simulink model "PID_CorSys_Ctrl"  (R2018b)
settings: Solver=ode1  StartTime=0.0  StopTime=inf  FixedStep=0.01  RelTol=1e-3  EnableMultiTasking=on
libraries: gtbox x3
settings Model: SimulationMode=external  ExtModeTrigDuration=200000  Creator=David  LastModifiedBy=optiplex3060
settings DataIOCC: LimitDataPoints=on  SaveFormat=Array  SignalLoggingSaveFormat=ModelDataLogs
settings OptimizationCC: ExpressionDepthLimit=2147483647
settings DebuggingCC: UnderspecifiedInitializationDetection=Classic  MergeDetectMultiDrivingBlocksExec=none  SolverPrmCheckMsg=warning  FcnCallInpInsideContextMsg=warning  StateNameClashWarn=warning  SFUnexpectedBacktrackingDiag=warning  SFNoUnconditionalDefaultTransitionDiag=warning  SFExecutionAtInitializationDiag=none
settings ModelReferenceCC: PropagateSignalLabelsOutOfModel=off
settings SFSimCC: SimUseLocalCustomCode=off
settings RTWCC: SystemTargetFile=sldrt.tlc  TemplateMakefile=sldrt.tmf  Description=Simulink Desktop Real-Time  RTWUseLocalCustomCode=off  RTWCompilerOptimization=on
settings CodeAppCC: MaxIdLength=95  StateflowObjectComments=on
settings SimulinkDesktopRealTimeCC: TargetPreCompLibLocation=E:\Program Files\MATLAB\R2018b\toolbox\sldrt\lib\win64  TargetLangStandard=C89/C90 (ANSI)  SupportVariableSizeSignals=off  PreserveStateflowLocalDataDimensions=off
settings ConfigComp: CovMetricSettings=dw  CovHtmlReporting=on  CovSaveCumulativeToWorkspaceVar=on  CovSaveSingleToWorkspaceVar=on  CovExternalEMLEnable=off

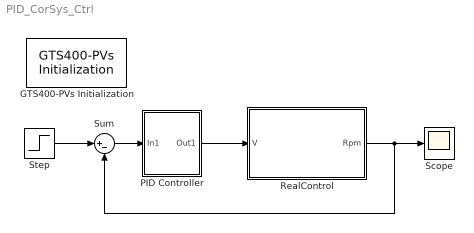
== system PID_CorSys_Ctrl ==
  GTS400-PVs Initialization : gtbox/GTS-400-PV Function Blocks/GTS400-PVs Initialization  Priority=0  open=0  mode=0  servo=[0 1 0 0]  aft=[0 0 0 0]  pid1=[1 0 0]  pid2=[1 0 0]  pid3=[1 0 0]  pid4=[1 0 0]  enc1=off  enc2=on  enc3=off  enc4=off  lmt1=off  lmt2=off  lmt3=off  lmt4=off  cdno=2
      settings: SourceProductName=Googol Education Products v2.0
  PID Controller : Subsystem  mask{Kp=0.4, Ki=4.5, Kd=0}
      mask help: PID Controller.
      mask Help: PID Controller.
      mask Display: disp('PID')
  RealControl : Subsystem
      mask Display:
      | disp('Motor');
      | port_label('input', 1, 'RpmIn');
      | port_label('Output',1, 'RpmOut');
  Scope : Scope
  Step : Step  After=2000  SampleTime=0
  Sum : Sum  Inputs=|+-
  wires:
  RealControl/1(Rpm) -> Scope/1, Sum/2
  Sum/1 -> PID Controller/1(In1)
  PID Controller/1(Out1) -> RealControl/1(V)
  Step/1 -> Sum/1

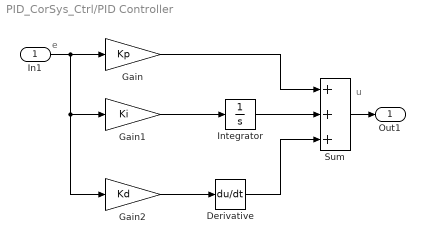
== system PID_CorSys_Ctrl/PID Controller ==
  note: u
  note: e
  In1 : Inport
  Derivative : Derivative
  Gain : Gain  Gain=Kp  SaturateOnIntegerOverflow=on  OutDataTypeStr=Inherit: Same as input  ParamDataTypeStr=Inherit: Same as input
  Gain1 : Gain  Gain=Ki  SaturateOnIntegerOverflow=on  OutDataTypeStr=Inherit: Same as input  ParamDataTypeStr=Inherit: Same as input
  Gain2 : Gain  Gain=Kd  SaturateOnIntegerOverflow=on  OutDataTypeStr=Inherit: Same as input  ParamDataTypeStr=Inherit: Same as input
  Integrator : Integrator
  Sum : Sum  Inputs=+++  SaturateOnIntegerOverflow=on  InputSameDT=on  OutDataTypeStr=Inherit: Same as first input
  Out1 : Outport
  wires:
  Integrator/1 -> Sum/2
  In1/1 -> Gain/1, Gain1/1, Gain2/1
  Sum/1 -> Out1/1
  Derivative/1 -> Sum/3
  Gain2/1 -> Derivative/1
  Gain1/1 -> Integrator/1
  Gain/1 -> Sum/1

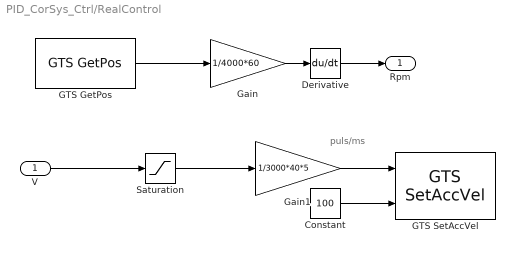
== system PID_CorSys_Ctrl/RealControl ==
  note: puls/ms
  V : Inport
  Constant : Constant  Value=100
  Derivative : Derivative
  GTS GetPos : gtbox/GTS-400-PV Function Blocks/GTS GetPos  axis=2
      settings: SourceProductName=Googol Education Products v2.0
  GTS SetAccVel : gtbox/GTS-400-PV Function Blocks/GTS SetAccVel  Axis=2  vel=0.1  pos=250000000000
      settings: SourceProductName=Googol Education Products v2.0
  Gain : Gain  Gain=1/4000*60
  Gain1 : Gain  Gain=1/3000*40*5
  Saturation : Saturate  UpperLimit=3000  LowerLimit=-3000
  Rpm : Outport
  wires:
  Constant/1 -> GTS SetAccVel/2
  Gain/1 -> Derivative/1
  Derivative/1 -> Rpm/1
  GTS GetPos/1 -> Gain/1
  Gain1/1 -> GTS SetAccVel/1
  Saturation/1 -> Gain1/1
  V/1 -> Saturation/1
